simulink model "mod_packet"  (R2023b)
settings: Solver=ode5  StartTime=0.0  StopTime=1  RelTol=1e-3
undefined symbols (not defined in the file or in its folder): Serial_Port, Standard_Devices
libraries: sldrtlib x3
settings Model: Creator=farfar  LastModifiedBy=farfar
settings HardwareCC: ProdBitPerLong=64  ProdHWDeviceType=Intel->x86-64 (Linux 64)
settings RTWCC: Description=Simulink Desktop Real-Time  SystemTargetFile=sldrt.tlc  TemplateMakefile=sldrt.tmf  RTWCompilerOptimization=on
settings CodeAppCC: MaxIdLength=95
settings SimulinkDesktopRealTimeCC: TargetLibSuffix=_sldrt.a  TargetPreCompLibLocation=C:\Program Files\MATLAB\R2023b\toolbox\sldrt\lib\win64

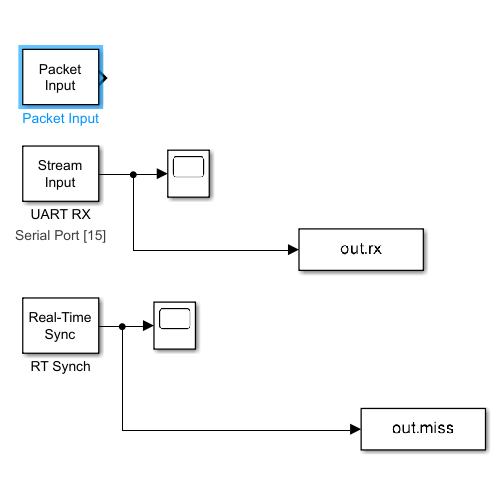
[thumbnail: Simulink's stored preview of the top-level diagram]
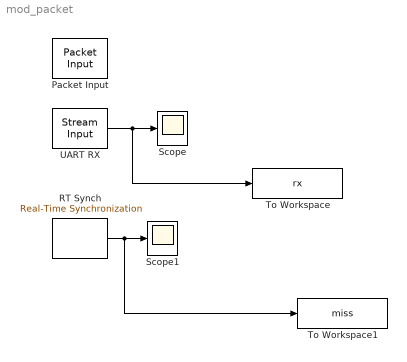
== system mod_packet ==
  Packet Input : sldrtlib/Packet Input  SampleTime=0.1  MaxMissedTicks=10  ShowMissedTicks=off  YieldWhenWaiting=off  DrvAddress=0  DrvOptions=0  PacketSize=32  DataTypes='4*double'  ShowReady=off  ShowError=off  PacketID=1  ByteOrder=1  ShowTimestamp=off
  RT Synch : sldrtlib/Real-Time Synchronization  SampleTime=0.004  MaxMissedTicks=10000  ShowMissedTicks=on  YieldWhenWaiting=off
  Scope : Scope
  Scope1 : Scope
  To Workspace : ToWorkspace  VariableName=rx  SaveFormat=Structure With Time  SampleTime=-1
  To Workspace1 : ToWorkspace  VariableName=miss  SaveFormat=Structure With Time  SampleTime=-1
  UART RX : sldrtlib/Stream Input  SampleTime=0.004  MaxMissedTicks=10000  ShowMissedTicks=off  YieldWhenWaiting=off  DrvName=Standard_Devices/Serial_Port  DrvAddress=15  DrvOptions=[115200 8 0 0 0 0 0 0]  DataTypes={'uint32'}  FormatString='%d'  Terminator={'\n'}  ShowReady=off  ShowError=off
      settings: AttributesFormatString=Serial Port [15]
  wires:
  RT Synch/1 -> To Workspace1/1, Scope1/1
  UART RX/1 -> To Workspace/1, Scope/1
